simulink model "Tarea4_base"  (R2022b)
settings: Solver=FixedStepDiscrete  StartTime=0.0  StopTime=Tsim  FixedStep=Ts  RelTol=1e-3
values from neighbouring files (symbols this model uses):
  a_adj = ones(3)    [P1.m]
  a_Costo_1 = 0.444    [Tarea4_init.m]
  a_Costo_2 = 0.264    [Tarea4_init.m]
  a_Costo_3 = 0.5    [Tarea4_init.m]
  b_Costo_1 = 0.111    [Tarea4_init.m]
  b_Costo_2 = 0.067    [Tarea4_init.m]
  b_Costo_3 = 0.125    [Tarea4_init.m]
  e_DG1 = 0    [Tarea4_init.m]
  e_DG2 = 0    [Tarea4_init.m]
  e_DG3 = 0    [Tarea4_init.m]
  e_droop = 0    [Tarea4_init.m]
  e_secondary = 100    [Tarea4_init.m]
  fc = 1    [Tarea4_init.m]
  Kii = Lf*wni*wni    (= 8389.16374093)    [Tarea4_init.m]
  Kiv = wnv*wnv*Cf*10    (= 69.0872308076)    [Tarea4_init.m]
  Kpi = 2*zeta*wni*Lf    (= 4.27256600888)    [Tarea4_init.m]
  Kpv = 2*zeta*wnv*Cf*10    (= 0.351858377202)    [Tarea4_init.m]
  Mdc_1 = -30/Pmax_1    (= -0.012)    [Tarea4_init.m]
  Mdc_2 = -30/Pmax_2    (= -0.012)    [Tarea4_init.m]
  Mdc_3 = -30/Pmax_3    (= -0.012)    [Tarea4_init.m]
  mpc_sample_time = 3    [P1.m]
  Pmax_1 = 2500    [Tarea4_init.m]
  Pmax_2 = Pmax_1    (= 2500)    [Tarea4_init.m]
  Pmax_3 = Pmax_1    (= 2500)    [Tarea4_init.m]
  Rl_1_DC = 100    [Tarea4_init.m]
  Rl_2_DC = 100    [Tarea4_init.m]
  Rl_3_DC = 125    [Tarea4_init.m]
  tau = 1*mpc_sample_time    (= 3)    [P1.m]
  Ts = 1/16e3    (= 6.25e-05)    [Tarea4_init.m]
  V0_dc = 400    [Tarea4_init.m]    (also in dmpc.m = parametros(6))
  Vmax_dc = V0_dc+5    (= 405)    [Tarea4_init.m]    (also in dmpc.m = parametros(8))
  Vmin_dc = V0_dc-5    (= 395)    [Tarea4_init.m]    (also in dmpc.m = parametros(7))
undefined symbols (not defined in the file or in its folder): plecs
libraries: slpidlib x6
settings Model: Creator=matib  LastModifiedBy=zanar
settings DebuggingCC: UnconnectedInputMsg=warning  UnconnectedOutputMsg=warning  UnconnectedLineMsg=warning  SFMachineParentedDataDiag=warning  UnderSpecifiedDimensionMsg=warning
settings ModelReferenceCC: EnableRefExpFcnMdlSchedulingChecks=on

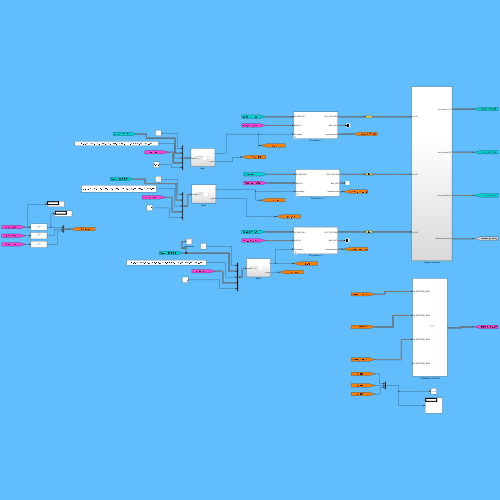
[thumbnail: Simulink's stored preview of the top-level diagram]
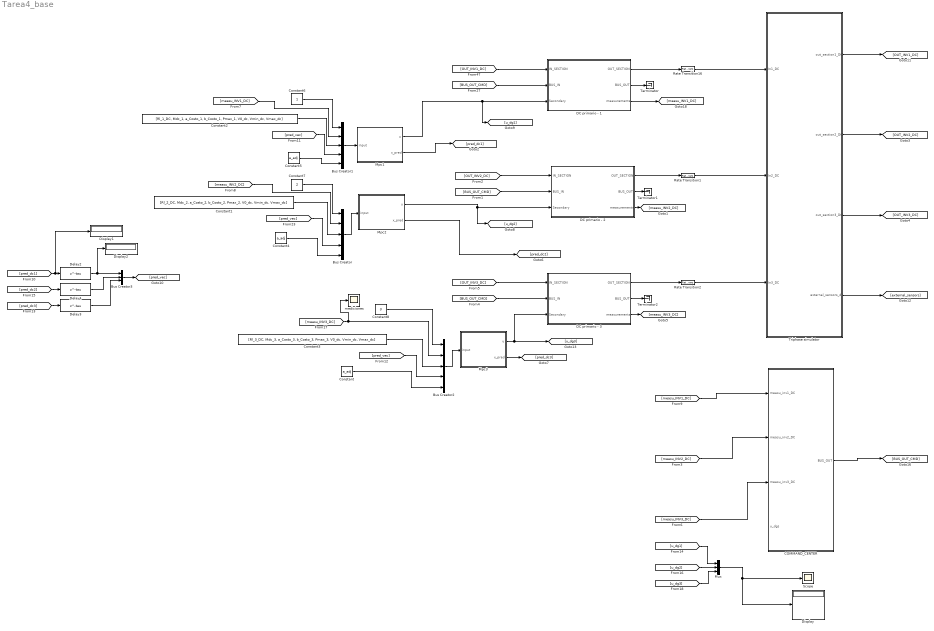
== system Tarea4_base ==
  Bus Creator : BusCreator  Inputs=5
  Bus Creator1 : BusCreator  Inputs=5
  Bus Creator2 : BusCreator  Inputs=5
  Bus Creator3 : BusCreator  Inputs=3
  COMMAND_CENTER : Subsystem
      mask Display:
      | port_label('input', 1, 'IN_SECTION_INV1');
      | port_label('input', 2, 'IN_SECTION_INV2');
      | port_label('input', 3, 'IN_SECTION_INV3');
      | port_label('input', 4, 'IN_SECTION_INV4');
      | 
      | port_label('input', 5, 'MEASUREMENT_INV1');
      | port_label('input', 6, 'MEASUREMENT_INV2');
      | port_label('input', 7, 'MEASUREMENT_INV3');
      | port_label('input', 8, 'MEASUREMENT_INV4');
      | 
      | port_label('input', 9, 'BUS_IN');
      | %port_label('input', 10, 'MEASUREMENT_SECONDARY');
      | 
      | port_label('output', 1, 'BUS_OUT');
  Constant : Constant  Value=a_adj
  Constant1 : Constant  Value=[Rl_2_DC, Mdc_2, a_Costo_2, b_Costo_2, Pmax_2, V0_dc, Vmin_dc, Vmax_dc]
  Constant2 : Constant  Value=[Rl_1_DC, Mdc_1, a_Costo_1, b_Costo_1, Pmax_1, V0_dc, Vmin_dc, Vmax_dc]
  Constant3 : Constant  Value=[Rl_3_DC, Mdc_3, a_Costo_3, b_Costo_3, Pmax_3, V0_dc, Vmin_dc, Vmax_dc]
  Constant4 : Constant  Value=a_adj
  Constant5 : Constant  Value=a_adj
  Constant6 : Constant
  Constant7 : Constant  Value=2
  Constant8 : Constant  Value=3
  DC primario - 1 : Subsystem  mask{Imax=2.5, Pmax=0, Tmax=0}
      mask prompts: Imax "Corriente Máxima"; Pmax "Potencia  Máxima"; Tmax "Temperatura  Máxima"
  DC primario - 2 : Subsystem  mask{Imax=2.5, Pmax=0, Tmax=0}
      mask prompts: Imax "Corriente Máxima"; Pmax "Potencia  Máxima"; Tmax "Temperatura  Máxima"
  DC primario - 3 : Subsystem  mask{Imax=2.5, Pmax=0, Tmax=0}
      mask prompts: Imax "Corriente Máxima"; Pmax "Potencia  Máxima"; Tmax "Temperatura  Máxima"
  Delay2 : Delay  DelayLength=tau
  Delay3 : Delay  DelayLength=tau
  Delay4 : Delay  DelayLength=tau
  Display : Display
  Display1 : Display
  Display2 : Display
  Mpc1 : Subsystem
  Mpc2 : Subsystem
  Mpc3 : Subsystem
  Mux : Mux  Inputs=3
  Rate Transition1 : RateTransition  OutPortSampleTime=Ts
  Rate Transition16 : RateTransition  OutPortSampleTime=Ts
  Rate Transition2 : RateTransition  OutPortSampleTime=Ts
  Scope : Scope
  Terminator : Terminator
  Terminator1 : Terminator
  Terminator2 : Terminator
  Triphase simulator : Subsystem
  mediciones : Scope
  wires:
  Triphase simulator/1(out_section1_DC) -> [OUT_INV1_DC]
  DC primario - 1/1(OUT_SECTION) -> Rate Transition16/1
  Rate Transition16/1 -> Triphase simulator/1(In1_DC)
  [OUT_INV1_DC] -> DC primario - 1/1(IN_SECTION)
  DC primario - 1/3(measurements) -> [measu_INV1_DC]
  [BUS_OUT_CMD] -> DC primario - 1/2(BUS_IN)
  [measu_INV1_DC] -> COMMAND_CENTER/1(measu_inv1_DC)
  COMMAND_CENTER/1(BUS_OUT) -> [BUS_OUT_CMD]
  DC primario - 2/3(measurements) -> [measu_INV2_DC]
  [OUT_INV2_DC] -> DC primario - 2/1(IN_SECTION)
  [BUS_OUT_CMD] -> DC primario - 2/2(BUS_IN)
  DC primario - 2/1(OUT_SECTION) -> Rate Transition1/1
  Rate Transition1/1 -> Triphase simulator/2(In2_DC)
  Triphase simulator/2(out_section2_DC) -> [OUT_INV2_DC]
  [measu_INV2_DC] -> COMMAND_CENTER/2(measu_inv2_DC)
  Triphase simulator/3(out_section3_DC) -> [OUT_INV3_DC]
  Rate Transition2/1 -> Triphase simulator/3(In3_DC)
  DC primario - 3/3(measurements) -> [measu_INV3_DC]
  DC primario - 3/1(OUT_SECTION) -> Rate Transition2/1
  [OUT_INV3_DC] -> DC primario - 3/1(IN_SECTION)
  [BUS_OUT_CMD] -> DC primario - 3/2(BUS_IN)
  [measu_INV3_DC] -> COMMAND_CENTER/3(measu_inv3_DC)
  DC primario - 1/2(BUS_OUT) -> Terminator/1
  DC primario - 2/2(BUS_OUT) -> Terminator1/1
  DC primario - 3/2(BUS_OUT) -> Terminator2/1
  Triphase simulator/4(external_sensors_dc) -> [external_sensors]
  [pred_dc1] -> Display1/1, Delay2/1
  [pred_dc3] -> Delay3/1
  [pred_dc2] -> Delay4/1
  Delay4/1 -> Bus Creator3/2
  Delay3/1 -> Bus Creator3/3
  [pred_vec] -> Bus Creator/4
  Constant1/1 -> Bus Creator/3
  Constant7/1 -> Bus Creator/1
  [measu_INV2_DC] -> Bus Creator/2
  [pred_vec] -> Bus Creator1/4
  [measu_INV1_DC] -> Bus Creator1/2
  Constant2/1 -> Bus Creator1/3
  Constant6/1 -> Bus Creator1/1
  [pred_vec] -> Bus Creator2/4
  Constant8/1 -> Bus Creator2/1
  Constant3/1 -> Bus Creator2/3
  Constant/1 -> Bus Creator2/5
  Constant4/1 -> Bus Creator/5
  Bus Creator3/1 -> [pred_vec]
  Mpc3/1(u) -> [u_dg3], DC primario - 3/3(Secondary)
  Bus Creator2/1 -> Mpc3/1(input)
  [measu_INV3_DC] -> mediciones/1, Bus Creator2/2
  Mpc1/2(x_pred) -> [pred_dc1]
  Mpc1/1(u) -> [u_dg1], DC primario - 1/3(Secondary)
  Bus Creator1/1 -> Mpc1/1(input)
  Bus Creator/1 -> Mpc2/1(input)
  Mpc2/1(u) -> [u_dg2], DC primario - 2/3(Secondary)
  Mpc2/2(x_pred) -> [pred_dc2]
  Mpc3/2(x_pred) -> [pred_dc3]
  Constant5/1 -> Bus Creator1/5
  [u_dg1] -> Mux/1
  [u_dg2] -> Mux/2
  [u_dg3] -> Mux/3
  Mux/1 -> Scope/1, Display/1
  Delay2/1 -> Display2/1, Bus Creator3/1

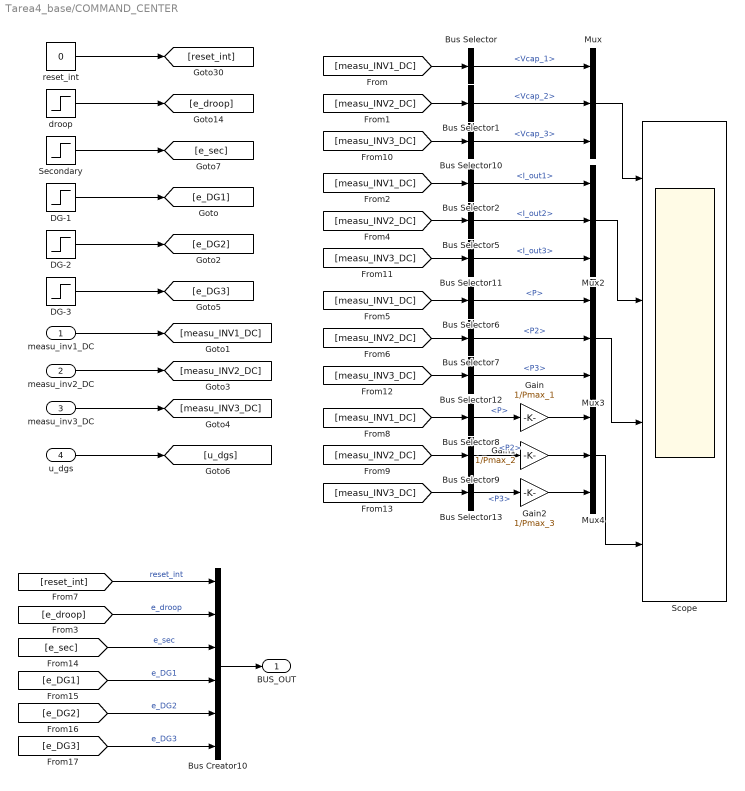
== system Tarea4_base/COMMAND_CENTER ==
  measu_inv1_DC : Inport
  measu_inv2_DC : Inport  Port=2
  measu_inv3_DC : Inport  Port=3
  u_dgs : Inport  Port=4
  Bus Creator10 : BusCreator  Inputs=6
  Bus Selector : BusSelector  OutputSignals=Vcap_1
  Bus Selector1 : BusSelector  OutputSignals=Vcap_2
  Bus Selector10 : BusSelector  OutputSignals=Vcap_3
  Bus Selector11 : BusSelector  OutputSignals=I_out3
  Bus Selector12 : BusSelector  OutputSignals=P3
  Bus Selector13 : BusSelector  OutputSignals=P3
  Bus Selector2 : BusSelector  OutputSignals=I_out1
  Bus Selector5 : BusSelector  OutputSignals=I_out2
  Bus Selector6 : BusSelector  OutputSignals=P
  Bus Selector7 : BusSelector  OutputSignals=P2
  Bus Selector8 : BusSelector  OutputSignals=P
  Bus Selector9 : BusSelector  OutputSignals=P2
  DG-1 : Step  Time=e_DG1  SampleTime=0
  DG-2 : Step  Time=e_DG2  SampleTime=0
  DG-3 : Step  Time=e_DG3  SampleTime=0
  Gain : Gain  Gain=1/Pmax_1
  Gain1 : Gain  Gain=1/Pmax_2
  Gain2 : Gain  Gain=1/Pmax_3
  Mux{,2..4} (4 alike) : Mux  Inputs=3
  Scope : Scope  NumInputPorts=4
  Secondary : Step  Time=e_secondary  SampleTime=0
  droop : Step  Time=e_droop  SampleTime=0
  reset_int : Constant  Value=0  OutDataTypeStr=boolean  SampleTime=Ts
  BUS_OUT : Outport
  wires:
  Bus Creator10/1 -> BUS_OUT/1
  [reset_int] -> Bus Creator10/1  "reset_int"
  reset_int/1 -> [reset_int]
  droop/1 -> [e_droop]
  measu_inv1_DC/1 -> [measu_INV1_DC]
  [e_droop] -> Bus Creator10/2  "e_droop"
  measu_inv2_DC/1 -> [measu_INV2_DC]
  [measu_INV1_DC] -> Bus Selector/1
  [measu_INV2_DC] -> Bus Selector1/1
  Bus Selector1/1 -> Mux/2  "<Vcap_2>"
  Bus Selector/1 -> Mux/1  "<Vcap_1>"
  Bus Selector2/1 -> Mux2/1  "<I_out1>"
  [measu_INV2_DC] -> Bus Selector5/1
  [measu_INV1_DC] -> Bus Selector2/1
  Bus Selector5/1 -> Mux2/2  "<I_out2>"
  [measu_INV1_DC] -> Bus Selector6/1
  Bus Selector7/1 -> Mux3/2  "<P2>"
  [measu_INV2_DC] -> Bus Selector7/1
  Bus Selector6/1 -> Mux3/1  "<P>"
  Mux3/1 -> Scope/3
  Mux2/1 -> Scope/2
  Mux/1 -> Scope/1
  [measu_INV1_DC] -> Bus Selector8/1
  [measu_INV2_DC] -> Bus Selector9/1
  Bus Selector9/1 -> Gain1/1  "<P2>"
  Mux4/1 -> Scope/4
  Bus Selector8/1 -> Gain/1  "<P>"
  Gain/1 -> Mux4/1
  Gain1/1 -> Mux4/2
  measu_inv3_DC/1 -> [measu_INV3_DC]
  Bus Selector10/1 -> Mux/3  "<Vcap_3>"
  [measu_INV3_DC] -> Bus Selector10/1
  [measu_INV3_DC] -> Bus Selector11/1
  Bus Selector11/1 -> Mux2/3  "<I_out3>"
  [measu_INV3_DC] -> Bus Selector12/1
  Bus Selector12/1 -> Mux3/3  "<P3>"
  Bus Selector13/1 -> Gain2/1  "<P3>"
  Gain2/1 -> Mux4/3
  [measu_INV3_DC] -> Bus Selector13/1
  [e_sec] -> Bus Creator10/3  "e_sec"
  [e_DG1] -> Bus Creator10/4  "e_DG1"
  [e_DG2] -> Bus Creator10/5  "e_DG2"
  [e_DG3] -> Bus Creator10/6  "e_DG3"
  DG-1/1 -> [e_DG1]
  DG-2/1 -> [e_DG2]
  DG-3/1 -> [e_DG3]
  Secondary/1 -> [e_sec]
  u_dgs/1 -> [u_dgs]

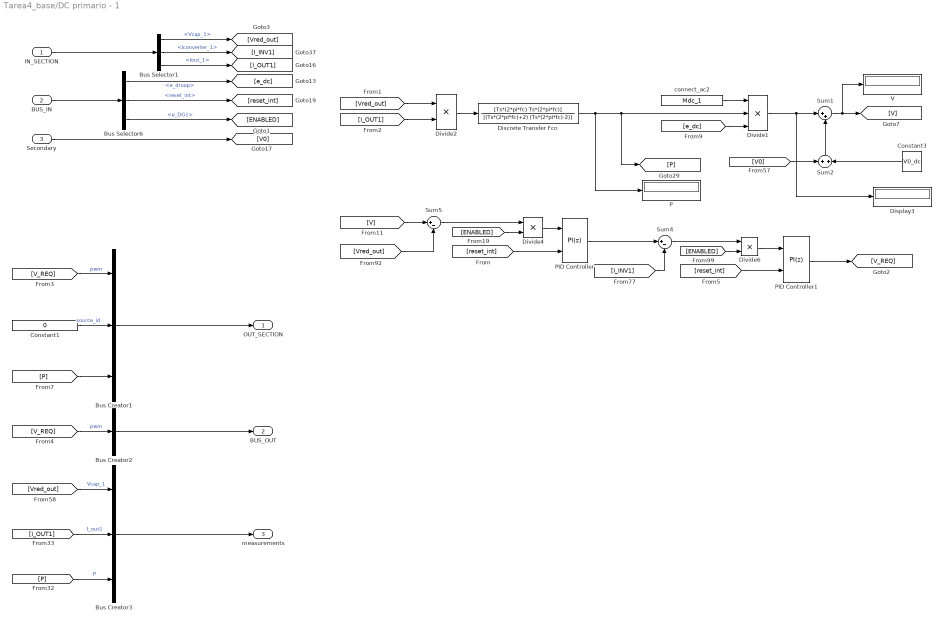
== system Tarea4_base/DC primario - 1 ==
  IN_SECTION : Inport
  BUS_IN : Inport  Port=2
  Secondary : Inport  Port=3
  Bus Creator1 : BusCreator  Inputs=3
  Bus Creator2 : BusCreator  Inputs=1
  Bus Creator3 : BusCreator  Inputs=3
  Bus Selector1 : BusSelector  OutputSignals=Vcap_1,Iconverter_1,Iout_1
  Bus Selector6 : BusSelector  OutputSignals=e_droop,reset_int,e_DG1
  Constant1 : Constant  Value=0  SampleTime=Ts
  Constant3 : Constant  Value=V0_dc  SampleTime=Ts
  Discrete Transfer Fcn : DiscreteTransferFcn  Numerator=[Ts*(2*pi*fc) Ts*(2*pi*fc)]  Denominator=[(Ts*(2*pi*fc)+2) (Ts*(2*pi*fc)-2)]  SampleTime=Ts
  Display3 : Display
  Divide1 : Product  Inputs=3
  Divide2 : Product
  Divide4 : Product  Inputs=**
  Divide6 : Product  Inputs=**
  P : Display
  PID Controller : slpidlib/PID Controller  Controller=PI  Form=Parallel  TimeDomain=Discrete-time  UseExternalTs=off  SampleTime=Ts  IntegratorMethod=Forward Euler  FilterMethod=Forward Euler  ControllerParametersSource=internal  P=Kpv  I=Kiv  UseKiTs=off  D=0  N=100  UseFilter=on  TunerSelectOption=Transfer Function Based (PID Tuner App)  InitialConditionSource=internal  InitialConditionForIntegrator=0  InitialConditionForFilter=0  DifferentiatorICPrevScaledInput=0  ExternalReset=rising  TrackingMode=off  Kt=1  LimitOutput=off  SatLimitsSource=internal  UpperSaturationLimit=500  LowerSaturationLimit=-500  LinearizeAsGain=on  AntiWindupMode=clamping  Kb=1  LimitIntegrator=off  UpperIntegratorSaturationLimit=inf  LowerIntegratorSaturationLimit=-inf  POutMin=[]  POutMax=[]  IOutMin=[]  IOutMax=[]  DOutMin=[]  DOutMax=[]  NOutMin=[]  NOutMax=[]  SumOutMin=[]  SumOutMax=[]  SaturationOutMin=[]  SaturationOutMax=[]  PParamMin=[]  PParamMax=[]  IParamMin=[]  IParamMax=[]  DParamMin=[]  DParamMax=[]  NParamMin=[]  NParamMax=[]  KbParamMin=[]  KbParamMax=[]  KtParamMin=[]  KtParamMax=[]  KbOutMin=[]  KbOutMax=[]  KtOutMin=[]  KtOutMax=[]  IntegratorOutMin=[]  IntegratorOutMax=[]  FilterOutMin=[]  FilterOutMax=[]  SumI1OutMin=[]  SumI1OutMax=[]  SumI2OutMin=[]  SumI2OutMax=[]  SumI3OutMin=[]  SumI3OutMax=[]  SumI4OutMin=[]  SumI4OutMax=[]  SumDOutMin=[]  SumDOutMax=[]  DifferentiatorOutMin=[]  DifferentiatorOutMax=[]  FilterDiffOutCoefMin=[]  FilterDiffOutCoefMax=[]  ReciprocalOutMin=[]  ReciprocalOutMax=[]  SumDenOutMin=[]  SumDenOutMax=[]  SumNumOutMin=[]  SumNumOutMax=[]  DivideOutMin=[]  DivideOutMax=[]  UdiffTsProdOutMin=[]  UdiffTsProdOutMax=[]  NTsProdOutMin=[]  NTsProdOutMax=[]  UintegralTsProdOutMin=[]  UintegralTsProdOutMax=[]  UngainTsProdOutMin=[]  UngainTsProdOutMax=[]  ClampingZeroOutDataTypeStr=Inherit: Inherit via back propagation  ClampingZeroOutMin=[]  ClampingZeroOutMax=[]  FilterDenConstantOutDataTypeStr=Inherit: Inherit via back propagation  FilterDenConstantOutMin=[]  FilterDenConstantOutMax=[]  PCopyOutDataTypeStr=Inherit: Inherit via back propagation  PCopyOutMin=[]  PCopyOutMax=[]  NCopyOutDataTypeStr=Inherit: Inherit via back propagation  NCopyOutMin=[]  NCopyOutMax=[]  IntegratorContinuousStateAttributes=''  IntegratorStateMustResolveToSignalObject=off  IntegratorRTWStateStorageClass=Auto  FilterContinuousStateAttributes=''  FilterStateMustResolveToSignalObject=off  FilterRTWStateStorageClass=Auto  ParallelPVariant=InternalParameters  IdealPVariant=Disabled  IVariant=InternalParameters  DVariant=Disabled  IntegratorVariant=Discrete  SatVariant=Disabled  AWVariant=Passthrough  PCopyVariant=Disabled  TRVariant=Disabled  FdbkBlocksVariant=Forward  IdealPFdbkVariant=Disabled  SatFdbkVariant=Disabled  DerivativeFilterVariant=Disabled  NVariant=Disabled  NCopyVariant=Disabled_SignalSpec  FilterICVariant=Disabled  IntegratorICVariant=InternalICs  ExternalResetVariant=ExternalReset  TRSumVariant=Passthrough  SumFdbkVariant=Disabled  SumVariant=Sum_PI  TsampFilterVariant=InternalTs  TsampNgainVariant=Passthrough  TsampIntegralVariant=Passthrough  ExternalSaturationOutDataTypeStr=Inherit: Same as second input
  PID Controller1 : slpidlib/PID Controller  Controller=PI  Form=Parallel  TimeDomain=Discrete-time  UseExternalTs=off  SampleTime=Ts  IntegratorMethod=Forward Euler  FilterMethod=Forward Euler  ControllerParametersSource=internal  P=Kpi  I=Kii  UseKiTs=off  D=0  N=100  UseFilter=on  TunerSelectOption=Transfer Function Based (PID Tuner App)  InitialConditionSource=internal  InitialConditionForIntegrator=0  InitialConditionForFilter=0  DifferentiatorICPrevScaledInput=0  ExternalReset=rising  TrackingMode=off  Kt=1  LimitOutput=off  SatLimitsSource=internal  UpperSaturationLimit=inf  LowerSaturationLimit=-inf  LinearizeAsGain=on  AntiWindupMode=none  Kb=1  LimitIntegrator=off  UpperIntegratorSaturationLimit=inf  LowerIntegratorSaturationLimit=-inf  POutMin=[]  POutMax=[]  IOutMin=[]  IOutMax=[]  DOutMin=[]  DOutMax=[]  NOutMin=[]  NOutMax=[]  SumOutMin=[]  SumOutMax=[]  SaturationOutMin=[]  SaturationOutMax=[]  PParamMin=[]  PParamMax=[]  IParamMin=[]  IParamMax=[]  DParamMin=[]  DParamMax=[]  NParamMin=[]  NParamMax=[]  KbParamMin=[]  KbParamMax=[]  KtParamMin=[]  KtParamMax=[]  KbOutMin=[]  KbOutMax=[]  KtOutMin=[]  KtOutMax=[]  IntegratorOutMin=[]  IntegratorOutMax=[]  FilterOutMin=[]  FilterOutMax=[]  SumI1OutMin=[]  SumI1OutMax=[]  SumI2OutMin=[]  SumI2OutMax=[]  SumI3OutMin=[]  SumI3OutMax=[]  SumI4OutMin=[]  SumI4OutMax=[]  SumDOutMin=[]  SumDOutMax=[]  DifferentiatorOutMin=[]  DifferentiatorOutMax=[]  FilterDiffOutCoefMin=[]  FilterDiffOutCoefMax=[]  ReciprocalOutMin=[]  ReciprocalOutMax=[]  SumDenOutMin=[]  SumDenOutMax=[]  SumNumOutMin=[]  SumNumOutMax=[]  DivideOutMin=[]  DivideOutMax=[]  UdiffTsProdOutMin=[]  UdiffTsProdOutMax=[]  NTsProdOutMin=[]  NTsProdOutMax=[]  UintegralTsProdOutMin=[]  UintegralTsProdOutMax=[]  UngainTsProdOutMin=[]  UngainTsProdOutMax=[]  ClampingZeroOutDataTypeStr=Inherit: Inherit via back propagation  ClampingZeroOutMin=[]  ClampingZeroOutMax=[]  FilterDenConstantOutDataTypeStr=Inherit: Inherit via back propagation  FilterDenConstantOutMin=[]  FilterDenConstantOutMax=[]  PCopyOutDataTypeStr=Inherit: Inherit via back propagation  PCopyOutMin=[]  PCopyOutMax=[]  NCopyOutDataTypeStr=Inherit: Inherit via back propagation  NCopyOutMin=[]  NCopyOutMax=[]  IntegratorContinuousStateAttributes=''  IntegratorStateMustResolveToSignalObject=off  IntegratorRTWStateStorageClass=Auto  FilterContinuousStateAttributes=''  FilterStateMustResolveToSignalObject=off  FilterRTWStateStorageClass=Auto  ParallelPVariant=InternalParameters  IdealPVariant=Disabled  IVariant=InternalParameters  DVariant=Disabled  IntegratorVariant=Discrete  SatVariant=Disabled  AWVariant=Passthrough  PCopyVariant=Disabled  TRVariant=Disabled  FdbkBlocksVariant=Forward  IdealPFdbkVariant=Disabled  SatFdbkVariant=Disabled  DerivativeFilterVariant=Disabled  NVariant=Disabled  NCopyVariant=Disabled_SignalSpec  FilterICVariant=Disabled  IntegratorICVariant=InternalICs  ExternalResetVariant=ExternalReset  TRSumVariant=Passthrough  SumFdbkVariant=Disabled  SumVariant=Sum_PI  TsampFilterVariant=InternalTs  TsampNgainVariant=Passthrough  TsampIntegralVariant=Passthrough  ExternalSaturationOutDataTypeStr=Inherit: Same as second input
  Sum1 : Sum  Inputs=|++
  Sum2 : Sum  Inputs=+|+
  Sum4 : Sum  Inputs=|+-
  Sum5 : Sum  Inputs=|+-
  V : Display
  connect_ac2 : Constant  Value=Mdc_1  SampleTime=Ts
  OUT_SECTION : Outport  LockScale=on
  BUS_OUT : Outport  Port=2
  measurements : Outport  Port=3
  wires:
  connect_ac2/1 -> Divide1/1
  Sum1/1 -> V/1, [V]
  Divide1/1 -> Display3/1, Sum1/1
  [e_dc] -> Divide1/3
  IN_SECTION/1 -> Bus Selector1/1
  Bus Selector1/2 -> [I_INV1]  "<Iconverter_1>"
  Bus Selector1/3 -> [I_OUT1]  "<Iout_1>"
  Bus Creator2/1 -> BUS_OUT/1
  [V_REQ] -> Bus Creator2/1  "pwm"
  Constant1/1 -> Bus Creator1/2  "source_id"
  Bus Creator1/1 -> OUT_SECTION/1
  Bus Creator3/1 -> measurements/1
  [Vred_out] -> Bus Creator3/1  "Vcap_1"
  [V_REQ] -> Bus Creator1/1  "pwm"
  Sum2/1 -> Sum1/2
  [V0] -> Sum2/1
  [Vred_out] -> Divide2/1
  [I_OUT1] -> Divide2/2
  [P] -> Bus Creator3/3  "P"
  [I_OUT1] -> Bus Creator3/2  "I_out1"
  [P] -> Bus Creator1/3
  Divide2/1 -> Discrete Transfer Fcn/1
  Discrete Transfer Fcn/1 -> Divide1/2, [P], P/1
  Bus Selector1/1 -> [Vred_out]  "<Vcap_1>"
  [Vred_out] -> Sum5/2
  [ENABLED] -> Divide6/2
  [ENABLED] -> Divide4/2
  Sum5/1 -> Divide4/1
  Sum4/1 -> Divide6/1
  [reset_int] -> PID Controller/2
  [V] -> Sum5/1
  [I_INV1] -> Sum4/2
  [reset_int] -> PID Controller1/2
  Divide6/1 -> PID Controller1/1
  Divide4/1 -> PID Controller/1
  PID Controller/1 -> Sum4/1
  Constant3/1 -> Sum2/2
  PID Controller1/1 -> [V_REQ]
  Bus Selector6/2 -> [reset_int]  "<reset_int>"
  Bus Selector6/1 -> [e_dc]  "<e_droop>"
  BUS_IN/1 -> Bus Selector6/1
  Secondary/1 -> [V0]
  Bus Selector6/3 -> [ENABLED]  "<e_DG1>"

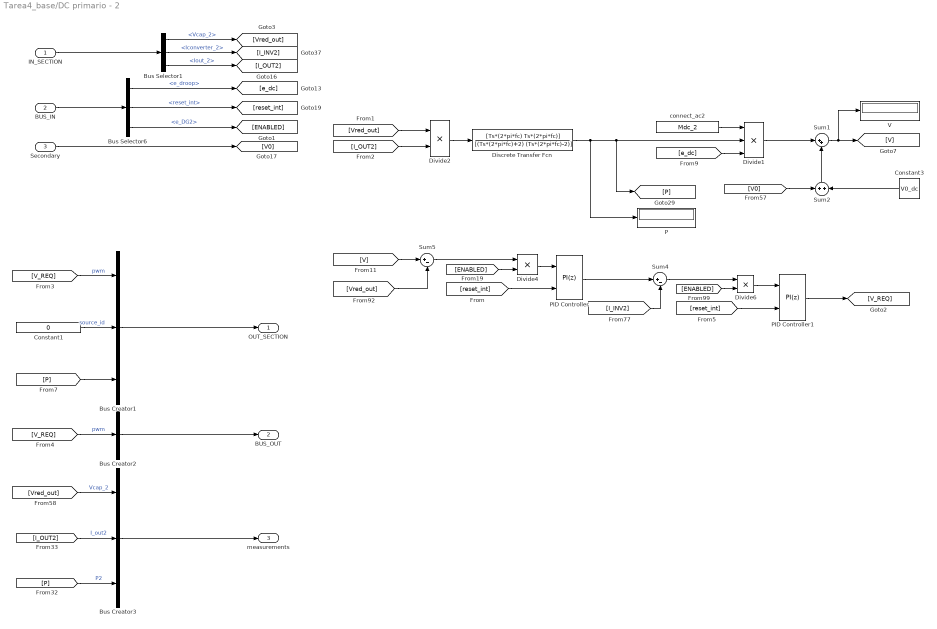
== system Tarea4_base/DC primario - 2 ==
  IN_SECTION : Inport
  BUS_IN : Inport  Port=2
  Secondary : Inport  Port=3
  Bus Creator1 : BusCreator  Inputs=3
  Bus Creator2 : BusCreator  Inputs=1
  Bus Creator3 : BusCreator  Inputs=3
  Bus Selector1 : BusSelector  OutputSignals=Vcap_2,Iconverter_2,Iout_2
  Bus Selector6 : BusSelector  OutputSignals=e_droop,reset_int,e_DG2
  Constant1 : Constant  Value=0  SampleTime=Ts
  Constant3 : Constant  Value=V0_dc  SampleTime=Ts
  Discrete Transfer Fcn : DiscreteTransferFcn  Numerator=[Ts*(2*pi*fc) Ts*(2*pi*fc)]  Denominator=[(Ts*(2*pi*fc)+2) (Ts*(2*pi*fc)-2)]  SampleTime=Ts
  Divide1 : Product  Inputs=3
  Divide2 : Product
  Divide4 : Product  Inputs=**
  Divide6 : Product  Inputs=**
  P : Display
  PID Controller : slpidlib/PID Controller  Controller=PI  Form=Parallel  TimeDomain=Discrete-time  UseExternalTs=off  SampleTime=Ts  IntegratorMethod=Forward Euler  FilterMethod=Forward Euler  ControllerParametersSource=internal  P=Kpv  I=Kiv  UseKiTs=off  D=0  N=100  UseFilter=on  TunerSelectOption=Transfer Function Based (PID Tuner App)  InitialConditionSource=internal  InitialConditionForIntegrator=0  InitialConditionForFilter=0  DifferentiatorICPrevScaledInput=0  ExternalReset=rising  TrackingMode=off  Kt=1  LimitOutput=off  SatLimitsSource=internal  UpperSaturationLimit=500  LowerSaturationLimit=-500  LinearizeAsGain=on  AntiWindupMode=clamping  Kb=1  LimitIntegrator=off  UpperIntegratorSaturationLimit=inf  LowerIntegratorSaturationLimit=-inf  POutMin=[]  POutMax=[]  IOutMin=[]  IOutMax=[]  DOutMin=[]  DOutMax=[]  NOutMin=[]  NOutMax=[]  SumOutMin=[]  SumOutMax=[]  SaturationOutMin=[]  SaturationOutMax=[]  PParamMin=[]  PParamMax=[]  IParamMin=[]  IParamMax=[]  DParamMin=[]  DParamMax=[]  NParamMin=[]  NParamMax=[]  KbParamMin=[]  KbParamMax=[]  KtParamMin=[]  KtParamMax=[]  KbOutMin=[]  KbOutMax=[]  KtOutMin=[]  KtOutMax=[]  IntegratorOutMin=[]  IntegratorOutMax=[]  FilterOutMin=[]  FilterOutMax=[]  SumI1OutMin=[]  SumI1OutMax=[]  SumI2OutMin=[]  SumI2OutMax=[]  SumI3OutMin=[]  SumI3OutMax=[]  SumI4OutMin=[]  SumI4OutMax=[]  SumDOutMin=[]  SumDOutMax=[]  DifferentiatorOutMin=[]  DifferentiatorOutMax=[]  FilterDiffOutCoefMin=[]  FilterDiffOutCoefMax=[]  ReciprocalOutMin=[]  ReciprocalOutMax=[]  SumDenOutMin=[]  SumDenOutMax=[]  SumNumOutMin=[]  SumNumOutMax=[]  DivideOutMin=[]  DivideOutMax=[]  UdiffTsProdOutMin=[]  UdiffTsProdOutMax=[]  NTsProdOutMin=[]  NTsProdOutMax=[]  UintegralTsProdOutMin=[]  UintegralTsProdOutMax=[]  UngainTsProdOutMin=[]  UngainTsProdOutMax=[]  ClampingZeroOutDataTypeStr=Inherit: Inherit via back propagation  ClampingZeroOutMin=[]  ClampingZeroOutMax=[]  FilterDenConstantOutDataTypeStr=Inherit: Inherit via back propagation  FilterDenConstantOutMin=[]  FilterDenConstantOutMax=[]  PCopyOutDataTypeStr=Inherit: Inherit via back propagation  PCopyOutMin=[]  PCopyOutMax=[]  NCopyOutDataTypeStr=Inherit: Inherit via back propagation  NCopyOutMin=[]  NCopyOutMax=[]  IntegratorContinuousStateAttributes=''  IntegratorStateMustResolveToSignalObject=off  IntegratorRTWStateStorageClass=Auto  FilterContinuousStateAttributes=''  FilterStateMustResolveToSignalObject=off  FilterRTWStateStorageClass=Auto  ParallelPVariant=InternalParameters  IdealPVariant=Disabled  IVariant=InternalParameters  DVariant=Disabled  IntegratorVariant=Discrete  SatVariant=Disabled  AWVariant=Passthrough  PCopyVariant=Disabled  TRVariant=Disabled  FdbkBlocksVariant=Forward  IdealPFdbkVariant=Disabled  SatFdbkVariant=Disabled  DerivativeFilterVariant=Disabled  NVariant=Disabled  NCopyVariant=Disabled_SignalSpec  FilterICVariant=Disabled  IntegratorICVariant=InternalICs  ExternalResetVariant=ExternalReset  TRSumVariant=Passthrough  SumFdbkVariant=Disabled  SumVariant=Sum_PI  TsampFilterVariant=InternalTs  TsampNgainVariant=Passthrough  TsampIntegralVariant=Passthrough  ExternalSaturationOutDataTypeStr=Inherit: Same as second input
  PID Controller1 : slpidlib/PID Controller  Controller=PI  Form=Parallel  TimeDomain=Discrete-time  UseExternalTs=off  SampleTime=Ts  IntegratorMethod=Forward Euler  FilterMethod=Forward Euler  ControllerParametersSource=internal  P=Kpi  I=Kii  UseKiTs=off  D=0  N=100  UseFilter=on  TunerSelectOption=Transfer Function Based (PID Tuner App)  InitialConditionSource=internal  InitialConditionForIntegrator=0  InitialConditionForFilter=0  DifferentiatorICPrevScaledInput=0  ExternalReset=rising  TrackingMode=off  Kt=1  LimitOutput=off  SatLimitsSource=internal  UpperSaturationLimit=inf  LowerSaturationLimit=-inf  LinearizeAsGain=on  AntiWindupMode=none  Kb=1  LimitIntegrator=off  UpperIntegratorSaturationLimit=inf  LowerIntegratorSaturationLimit=-inf  POutMin=[]  POutMax=[]  IOutMin=[]  IOutMax=[]  DOutMin=[]  DOutMax=[]  NOutMin=[]  NOutMax=[]  SumOutMin=[]  SumOutMax=[]  SaturationOutMin=[]  SaturationOutMax=[]  PParamMin=[]  PParamMax=[]  IParamMin=[]  IParamMax=[]  DParamMin=[]  DParamMax=[]  NParamMin=[]  NParamMax=[]  KbParamMin=[]  KbParamMax=[]  KtParamMin=[]  KtParamMax=[]  KbOutMin=[]  KbOutMax=[]  KtOutMin=[]  KtOutMax=[]  IntegratorOutMin=[]  IntegratorOutMax=[]  FilterOutMin=[]  FilterOutMax=[]  SumI1OutMin=[]  SumI1OutMax=[]  SumI2OutMin=[]  SumI2OutMax=[]  SumI3OutMin=[]  SumI3OutMax=[]  SumI4OutMin=[]  SumI4OutMax=[]  SumDOutMin=[]  SumDOutMax=[]  DifferentiatorOutMin=[]  DifferentiatorOutMax=[]  FilterDiffOutCoefMin=[]  FilterDiffOutCoefMax=[]  ReciprocalOutMin=[]  ReciprocalOutMax=[]  SumDenOutMin=[]  SumDenOutMax=[]  SumNumOutMin=[]  SumNumOutMax=[]  DivideOutMin=[]  DivideOutMax=[]  UdiffTsProdOutMin=[]  UdiffTsProdOutMax=[]  NTsProdOutMin=[]  NTsProdOutMax=[]  UintegralTsProdOutMin=[]  UintegralTsProdOutMax=[]  UngainTsProdOutMin=[]  UngainTsProdOutMax=[]  ClampingZeroOutDataTypeStr=Inherit: Inherit via back propagation  ClampingZeroOutMin=[]  ClampingZeroOutMax=[]  FilterDenConstantOutDataTypeStr=Inherit: Inherit via back propagation  FilterDenConstantOutMin=[]  FilterDenConstantOutMax=[]  PCopyOutDataTypeStr=Inherit: Inherit via back propagation  PCopyOutMin=[]  PCopyOutMax=[]  NCopyOutDataTypeStr=Inherit: Inherit via back propagation  NCopyOutMin=[]  NCopyOutMax=[]  IntegratorContinuousStateAttributes=''  IntegratorStateMustResolveToSignalObject=off  IntegratorRTWStateStorageClass=Auto  FilterContinuousStateAttributes=''  FilterStateMustResolveToSignalObject=off  FilterRTWStateStorageClass=Auto  ParallelPVariant=InternalParameters  IdealPVariant=Disabled  IVariant=InternalParameters  DVariant=Disabled  IntegratorVariant=Discrete  SatVariant=Disabled  AWVariant=Passthrough  PCopyVariant=Disabled  TRVariant=Disabled  FdbkBlocksVariant=Forward  IdealPFdbkVariant=Disabled  SatFdbkVariant=Disabled  DerivativeFilterVariant=Disabled  NVariant=Disabled  NCopyVariant=Disabled_SignalSpec  FilterICVariant=Disabled  IntegratorICVariant=InternalICs  ExternalResetVariant=ExternalReset  TRSumVariant=Passthrough  SumFdbkVariant=Disabled  SumVariant=Sum_PI  TsampFilterVariant=InternalTs  TsampNgainVariant=Passthrough  TsampIntegralVariant=Passthrough  ExternalSaturationOutDataTypeStr=Inherit: Same as second input
  Sum1 : Sum  Inputs=|++
  Sum2 : Sum  Inputs=+|+
  Sum4 : Sum  Inputs=|+-
  Sum5 : Sum  Inputs=|+-
  V : Display
  connect_ac2 : Constant  Value=Mdc_2  SampleTime=Ts
  OUT_SECTION : Outport  LockScale=on
  BUS_OUT : Outport  Port=2
  measurements : Outport  Port=3
  wires:
  IN_SECTION/1 -> Bus Selector1/1
  Bus Selector1/2 -> [I_INV2]  "<Iconverter_2>"
  Bus Selector1/3 -> [I_OUT2]  "<Iout_2>"
  Bus Creator2/1 -> BUS_OUT/1
  [V_REQ] -> Bus Creator2/1  "pwm"
  Constant1/1 -> Bus Creator1/2  "source_id"
  Bus Creator1/1 -> OUT_SECTION/1
  Bus Creator3/1 -> measurements/1
  [Vred_out] -> Bus Creator3/1  "Vcap_2"
  [V_REQ] -> Bus Creator1/1  "pwm"
  [P] -> Bus Creator3/3  "P2"
  [I_OUT2] -> Bus Creator3/2  "I_out2"
  [P] -> Bus Creator1/3
  Bus Selector1/1 -> [Vred_out]  "<Vcap_2>"
  Divide2/1 -> Discrete Transfer Fcn/1
  connect_ac2/1 -> Divide1/1
  Sum1/1 -> V/1, [V]
  Discrete Transfer Fcn/1 -> Divide1/2, [P], P/1
  [V0] -> Sum2/1
  Divide1/1 -> Sum1/1
  Sum2/1 -> Sum1/2
  Constant3/1 -> Sum2/2
  [e_dc] -> Divide1/3
  [Vred_out] -> Divide2/1
  [I_OUT2] -> Divide2/2
  Sum4/1 -> Divide6/1
  [reset_int] -> PID Controller/2
  [ENABLED] -> Divide4/2
  Divide6/1 -> PID Controller1/1
  [Vred_out] -> Sum5/2
  Sum5/1 -> Divide4/1
  [reset_int] -> PID Controller1/2
  [I_INV2] -> Sum4/2
  Divide4/1 -> PID Controller/1
  [V] -> Sum5/1
  PID Controller1/1 -> [V_REQ]
  [ENABLED] -> Divide6/2
  PID Controller/1 -> Sum4/1
  Bus Selector6/2 -> [reset_int]  "<reset_int>"
  Bus Selector6/1 -> [e_dc]  "<e_droop>"
  Secondary/1 -> [V0]
  BUS_IN/1 -> Bus Selector6/1
  Bus Selector6/3 -> [ENABLED]  "<e_DG2>"

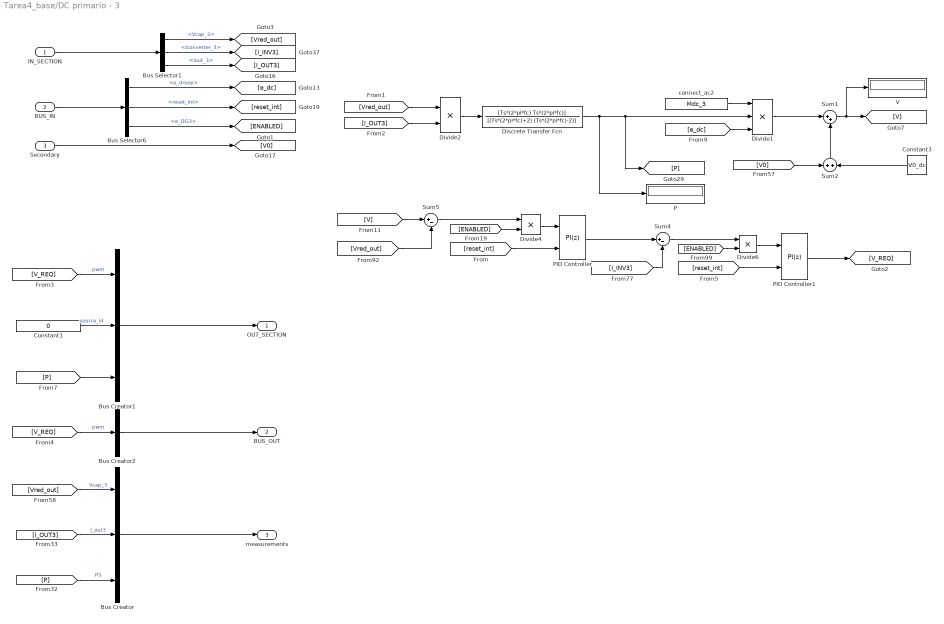
== system Tarea4_base/DC primario - 3 ==
  IN_SECTION : Inport
  BUS_IN : Inport  Port=2
  Secondary : Inport  Port=3
  Bus Creator : BusCreator  Inputs=3
  Bus Creator1 : BusCreator  Inputs=3
  Bus Creator2 : BusCreator  Inputs=1
  Bus Selector1 : BusSelector  OutputSignals=Vcap_3,Iconverter_3,Iout_3
  Bus Selector6 : BusSelector  OutputSignals=e_droop,reset_int,e_DG3
  Constant1 : Constant  Value=0  SampleTime=Ts
  Constant3 : Constant  Value=V0_dc  SampleTime=Ts
  Discrete Transfer Fcn : DiscreteTransferFcn  Numerator=[Ts*(2*pi*fc) Ts*(2*pi*fc)]  Denominator=[(Ts*(2*pi*fc)+2) (Ts*(2*pi*fc)-2)]  SampleTime=Ts
  Divide1 : Product  Inputs=3
  Divide2 : Product
  Divide4 : Product  Inputs=**
  Divide6 : Product  Inputs=**
  P : Display
  PID Controller : slpidlib/PID Controller  Controller=PI  Form=Parallel  TimeDomain=Discrete-time  UseExternalTs=off  SampleTime=Ts  IntegratorMethod=Forward Euler  FilterMethod=Forward Euler  ControllerParametersSource=internal  P=Kpv  I=Kiv  UseKiTs=off  D=0  N=100  UseFilter=on  TunerSelectOption=Transfer Function Based (PID Tuner App)  InitialConditionSource=internal  InitialConditionForIntegrator=0  InitialConditionForFilter=0  DifferentiatorICPrevScaledInput=0  ExternalReset=rising  TrackingMode=off  Kt=1  LimitOutput=off  SatLimitsSource=internal  UpperSaturationLimit=500  LowerSaturationLimit=-500  LinearizeAsGain=on  AntiWindupMode=clamping  Kb=1  LimitIntegrator=off  UpperIntegratorSaturationLimit=inf  LowerIntegratorSaturationLimit=-inf  POutMin=[]  POutMax=[]  IOutMin=[]  IOutMax=[]  DOutMin=[]  DOutMax=[]  NOutMin=[]  NOutMax=[]  SumOutMin=[]  SumOutMax=[]  SaturationOutMin=[]  SaturationOutMax=[]  PParamMin=[]  PParamMax=[]  IParamMin=[]  IParamMax=[]  DParamMin=[]  DParamMax=[]  NParamMin=[]  NParamMax=[]  KbParamMin=[]  KbParamMax=[]  KtParamMin=[]  KtParamMax=[]  KbOutMin=[]  KbOutMax=[]  KtOutMin=[]  KtOutMax=[]  IntegratorOutMin=[]  IntegratorOutMax=[]  FilterOutMin=[]  FilterOutMax=[]  SumI1OutMin=[]  SumI1OutMax=[]  SumI2OutMin=[]  SumI2OutMax=[]  SumI3OutMin=[]  SumI3OutMax=[]  SumI4OutMin=[]  SumI4OutMax=[]  SumDOutMin=[]  SumDOutMax=[]  DifferentiatorOutMin=[]  DifferentiatorOutMax=[]  FilterDiffOutCoefMin=[]  FilterDiffOutCoefMax=[]  ReciprocalOutMin=[]  ReciprocalOutMax=[]  SumDenOutMin=[]  SumDenOutMax=[]  SumNumOutMin=[]  SumNumOutMax=[]  DivideOutMin=[]  DivideOutMax=[]  UdiffTsProdOutMin=[]  UdiffTsProdOutMax=[]  NTsProdOutMin=[]  NTsProdOutMax=[]  UintegralTsProdOutMin=[]  UintegralTsProdOutMax=[]  UngainTsProdOutMin=[]  UngainTsProdOutMax=[]  ClampingZeroOutDataTypeStr=Inherit: Inherit via back propagation  ClampingZeroOutMin=[]  ClampingZeroOutMax=[]  FilterDenConstantOutDataTypeStr=Inherit: Inherit via back propagation  FilterDenConstantOutMin=[]  FilterDenConstantOutMax=[]  PCopyOutDataTypeStr=Inherit: Inherit via back propagation  PCopyOutMin=[]  PCopyOutMax=[]  NCopyOutDataTypeStr=Inherit: Inherit via back propagation  NCopyOutMin=[]  NCopyOutMax=[]  IntegratorContinuousStateAttributes=''  IntegratorStateMustResolveToSignalObject=off  IntegratorRTWStateStorageClass=Auto  FilterContinuousStateAttributes=''  FilterStateMustResolveToSignalObject=off  FilterRTWStateStorageClass=Auto  ParallelPVariant=InternalParameters  IdealPVariant=Disabled  IVariant=InternalParameters  DVariant=Disabled  IntegratorVariant=Discrete  SatVariant=Disabled  AWVariant=Passthrough  PCopyVariant=Disabled  TRVariant=Disabled  FdbkBlocksVariant=Forward  IdealPFdbkVariant=Disabled  SatFdbkVariant=Disabled  DerivativeFilterVariant=Disabled  NVariant=Disabled  NCopyVariant=Disabled_SignalSpec  FilterICVariant=Disabled  IntegratorICVariant=InternalICs  ExternalResetVariant=ExternalReset  TRSumVariant=Passthrough  SumFdbkVariant=Disabled  SumVariant=Sum_PI  TsampFilterVariant=InternalTs  TsampNgainVariant=Passthrough  TsampIntegralVariant=Passthrough  ExternalSaturationOutDataTypeStr=Inherit: Same as second input
  PID Controller1 : slpidlib/PID Controller  Controller=PI  Form=Parallel  TimeDomain=Discrete-time  UseExternalTs=off  SampleTime=Ts  IntegratorMethod=Forward Euler  FilterMethod=Forward Euler  ControllerParametersSource=internal  P=Kpi  I=Kii  UseKiTs=off  D=0  N=100  UseFilter=on  TunerSelectOption=Transfer Function Based (PID Tuner App)  InitialConditionSource=internal  InitialConditionForIntegrator=0  InitialConditionForFilter=0  DifferentiatorICPrevScaledInput=0  ExternalReset=rising  TrackingMode=off  Kt=1  LimitOutput=off  SatLimitsSource=internal  UpperSaturationLimit=inf  LowerSaturationLimit=-inf  LinearizeAsGain=on  AntiWindupMode=none  Kb=1  LimitIntegrator=off  UpperIntegratorSaturationLimit=inf  LowerIntegratorSaturationLimit=-inf  POutMin=[]  POutMax=[]  IOutMin=[]  IOutMax=[]  DOutMin=[]  DOutMax=[]  NOutMin=[]  NOutMax=[]  SumOutMin=[]  SumOutMax=[]  SaturationOutMin=[]  SaturationOutMax=[]  PParamMin=[]  PParamMax=[]  IParamMin=[]  IParamMax=[]  DParamMin=[]  DParamMax=[]  NParamMin=[]  NParamMax=[]  KbParamMin=[]  KbParamMax=[]  KtParamMin=[]  KtParamMax=[]  KbOutMin=[]  KbOutMax=[]  KtOutMin=[]  KtOutMax=[]  IntegratorOutMin=[]  IntegratorOutMax=[]  FilterOutMin=[]  FilterOutMax=[]  SumI1OutMin=[]  SumI1OutMax=[]  SumI2OutMin=[]  SumI2OutMax=[]  SumI3OutMin=[]  SumI3OutMax=[]  SumI4OutMin=[]  SumI4OutMax=[]  SumDOutMin=[]  SumDOutMax=[]  DifferentiatorOutMin=[]  DifferentiatorOutMax=[]  FilterDiffOutCoefMin=[]  FilterDiffOutCoefMax=[]  ReciprocalOutMin=[]  ReciprocalOutMax=[]  SumDenOutMin=[]  SumDenOutMax=[]  SumNumOutMin=[]  SumNumOutMax=[]  DivideOutMin=[]  DivideOutMax=[]  UdiffTsProdOutMin=[]  UdiffTsProdOutMax=[]  NTsProdOutMin=[]  NTsProdOutMax=[]  UintegralTsProdOutMin=[]  UintegralTsProdOutMax=[]  UngainTsProdOutMin=[]  UngainTsProdOutMax=[]  ClampingZeroOutDataTypeStr=Inherit: Inherit via back propagation  ClampingZeroOutMin=[]  ClampingZeroOutMax=[]  FilterDenConstantOutDataTypeStr=Inherit: Inherit via back propagation  FilterDenConstantOutMin=[]  FilterDenConstantOutMax=[]  PCopyOutDataTypeStr=Inherit: Inherit via back propagation  PCopyOutMin=[]  PCopyOutMax=[]  NCopyOutDataTypeStr=Inherit: Inherit via back propagation  NCopyOutMin=[]  NCopyOutMax=[]  IntegratorContinuousStateAttributes=''  IntegratorStateMustResolveToSignalObject=off  IntegratorRTWStateStorageClass=Auto  FilterContinuousStateAttributes=''  FilterStateMustResolveToSignalObject=off  FilterRTWStateStorageClass=Auto  ParallelPVariant=InternalParameters  IdealPVariant=Disabled  IVariant=InternalParameters  DVariant=Disabled  IntegratorVariant=Discrete  SatVariant=Disabled  AWVariant=Passthrough  PCopyVariant=Disabled  TRVariant=Disabled  FdbkBlocksVariant=Forward  IdealPFdbkVariant=Disabled  SatFdbkVariant=Disabled  DerivativeFilterVariant=Disabled  NVariant=Disabled  NCopyVariant=Disabled_SignalSpec  FilterICVariant=Disabled  IntegratorICVariant=InternalICs  ExternalResetVariant=ExternalReset  TRSumVariant=Passthrough  SumFdbkVariant=Disabled  SumVariant=Sum_PI  TsampFilterVariant=InternalTs  TsampNgainVariant=Passthrough  TsampIntegralVariant=Passthrough  ExternalSaturationOutDataTypeStr=Inherit: Same as second input
  Sum1 : Sum  Inputs=|++
  Sum2 : Sum  Inputs=+|+
  Sum4 : Sum  Inputs=|+-
  Sum5 : Sum  Inputs=|+-
  V : Display
  connect_ac2 : Constant  Value=Mdc_3  SampleTime=Ts
  OUT_SECTION : Outport  LockScale=on
  BUS_OUT : Outport  Port=2
  measurements : Outport  Port=3
  wires:
  IN_SECTION/1 -> Bus Selector1/1
  Bus Selector1/2 -> [I_INV3]  "<Iconverter_3>"
  Bus Selector1/3 -> [I_OUT3]  "<Iout_3>"
  Bus Creator2/1 -> BUS_OUT/1
  [V_REQ] -> Bus Creator2/1  "pwm"
  Constant1/1 -> Bus Creator1/2  "source_id"
  Bus Creator1/1 -> OUT_SECTION/1
  [Vred_out] -> Bus Creator/1  "Vcap_3"
  [V_REQ] -> Bus Creator1/1  "pwm"
  [P] -> Bus Creator/3  "P3"
  [I_OUT3] -> Bus Creator/2  "I_out3"
  [P] -> Bus Creator1/3
  Bus Selector1/1 -> [Vred_out]  "<Vcap_3>"
  Bus Creator/1 -> measurements/1
  Divide2/1 -> Discrete Transfer Fcn/1
  connect_ac2/1 -> Divide1/1
  Sum1/1 -> V/1, [V]
  Discrete Transfer Fcn/1 -> Divide1/2, [P], P/1
  [V0] -> Sum2/1
  Divide1/1 -> Sum1/1
  Sum2/1 -> Sum1/2
  Constant3/1 -> Sum2/2
  [e_dc] -> Divide1/3
  [Vred_out] -> Divide2/1
  [I_OUT3] -> Divide2/2
  Sum4/1 -> Divide6/1
  [reset_int] -> PID Controller/2
  [ENABLED] -> Divide4/2
  Divide6/1 -> PID Controller1/1
  [Vred_out] -> Sum5/2
  Sum5/1 -> Divide4/1
  [reset_int] -> PID Controller1/2
  [I_INV3] -> Sum4/2
  Divide4/1 -> PID Controller/1
  [V] -> Sum5/1
  PID Controller1/1 -> [V_REQ]
  [ENABLED] -> Divide6/2
  PID Controller/1 -> Sum4/1
  Bus Selector6/2 -> [reset_int]  "<reset_int>"
  Bus Selector6/1 -> [e_dc]  "<e_droop>"
  Secondary/1 -> [V0]
  BUS_IN/1 -> Bus Selector6/1
  Bus Selector6/3 -> [ENABLED]  "<e_DG3>"

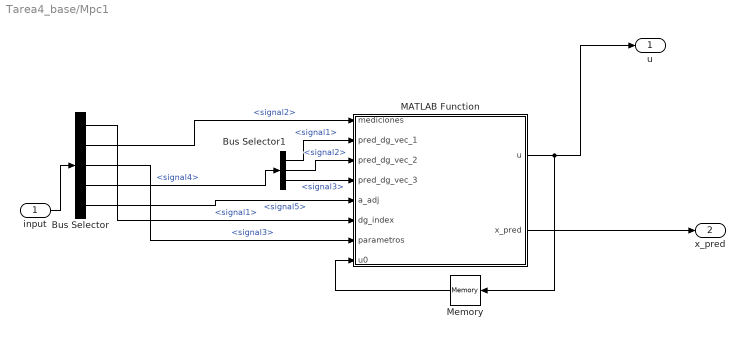
== system Tarea4_base/Mpc1 ==
  input : Inport
  Bus Selector : BusSelector  OutputSignals=signal1,signal2,signal3,signal4,signal5
  Bus Selector1 : BusSelector  OutputSignals=signal1,signal2,signal3
  MATLAB Function : MATLAB Function  TreatAsAtomicUnit=on  SystemSampleTime=mpc_sample_time
      settings: MinAlgLoopOccurrences=on
  Memory : Memory
  u : Outport
  x_pred : Outport  Port=2
  wires:
  MATLAB Function/1(u) -> Memory/1, u/1
  input/1 -> Bus Selector/1
  Bus Selector/2 -> MATLAB Function/1(mediciones)  "<signal2>"
  Bus Selector/4 -> Bus Selector1/1  "<signal4>"
  Bus Selector1/1 -> MATLAB Function/2(pred_dg_vec_1)  "<signal1>"
  Bus Selector1/2 -> MATLAB Function/3(pred_dg_vec_2)  "<signal2>"
  Bus Selector1/3 -> MATLAB Function/4(pred_dg_vec_3)  "<signal3>"
  MATLAB Function/2(x_pred) -> x_pred/1
  Bus Selector/1 -> MATLAB Function/6(dg_index)  "<signal1>"
  Bus Selector/3 -> MATLAB Function/7(parametros)  "<signal3>"
  Bus Selector/5 -> MATLAB Function/5(a_adj)  "<signal5>"
  Memory/1 -> MATLAB Function/8(u0)

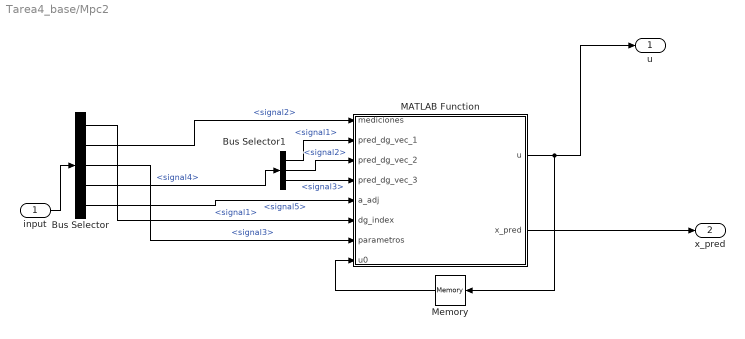
== system Tarea4_base/Mpc2 ==
  input : Inport
  Bus Selector : BusSelector  OutputSignals=signal1,signal2,signal3,signal4,signal5
  Bus Selector1 : BusSelector  OutputSignals=signal1,signal2,signal3
  MATLAB Function : MATLAB Function  TreatAsAtomicUnit=on  SystemSampleTime=mpc_sample_time
      settings: MinAlgLoopOccurrences=on
  Memory : Memory
  u : Outport
  x_pred : Outport  Port=2
  wires:
  Bus Selector/5 -> MATLAB Function/5(a_adj)  "<signal5>"
  Bus Selector/3 -> MATLAB Function/7(parametros)  "<signal3>"
  Bus Selector/1 -> MATLAB Function/6(dg_index)  "<signal1>"
  MATLAB Function/2(x_pred) -> x_pred/1
  Bus Selector1/3 -> MATLAB Function/4(pred_dg_vec_3)  "<signal3>"
  Bus Selector1/2 -> MATLAB Function/3(pred_dg_vec_2)  "<signal2>"
  Bus Selector1/1 -> MATLAB Function/2(pred_dg_vec_1)  "<signal1>"
  Bus Selector/4 -> Bus Selector1/1  "<signal4>"
  Bus Selector/2 -> MATLAB Function/1(mediciones)  "<signal2>"
  input/1 -> Bus Selector/1
  MATLAB Function/1(u) -> u/1, Memory/1
  Memory/1 -> MATLAB Function/8(u0)

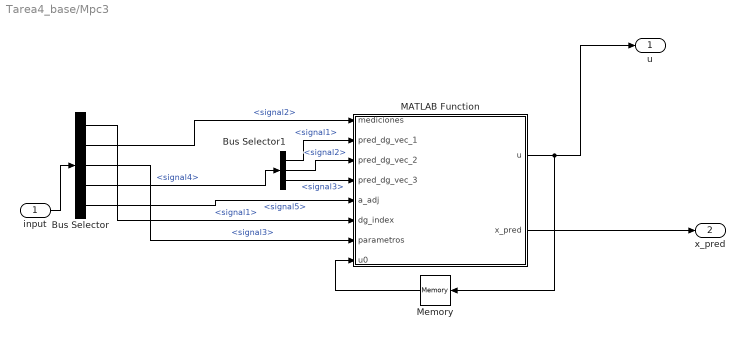
== system Tarea4_base/Mpc3 ==
  input : Inport
  Bus Selector : BusSelector  OutputSignals=signal1,signal2,signal3,signal4,signal5
  Bus Selector1 : BusSelector  OutputSignals=signal1,signal2,signal3
  MATLAB Function : MATLAB Function  TreatAsAtomicUnit=on  SystemSampleTime=mpc_sample_time
      settings: MinAlgLoopOccurrences=on
  Memory : Memory
  u : Outport
  x_pred : Outport  Port=2
  wires:
  MATLAB Function/1(u) -> Memory/1, u/1
  input/1 -> Bus Selector/1
  Bus Selector/2 -> MATLAB Function/1(mediciones)  "<signal2>"
  Bus Selector/4 -> Bus Selector1/1  "<signal4>"
  Bus Selector1/1 -> MATLAB Function/2(pred_dg_vec_1)  "<signal1>"
  Bus Selector1/2 -> MATLAB Function/3(pred_dg_vec_2)  "<signal2>"
  Bus Selector1/3 -> MATLAB Function/4(pred_dg_vec_3)  "<signal3>"
  MATLAB Function/2(x_pred) -> x_pred/1
  Bus Selector/1 -> MATLAB Function/6(dg_index)  "<signal1>"
  Bus Selector/3 -> MATLAB Function/7(parametros)  "<signal3>"
  Bus Selector/5 -> MATLAB Function/5(a_adj)  "<signal5>"
  Memory/1 -> MATLAB Function/8(u0)

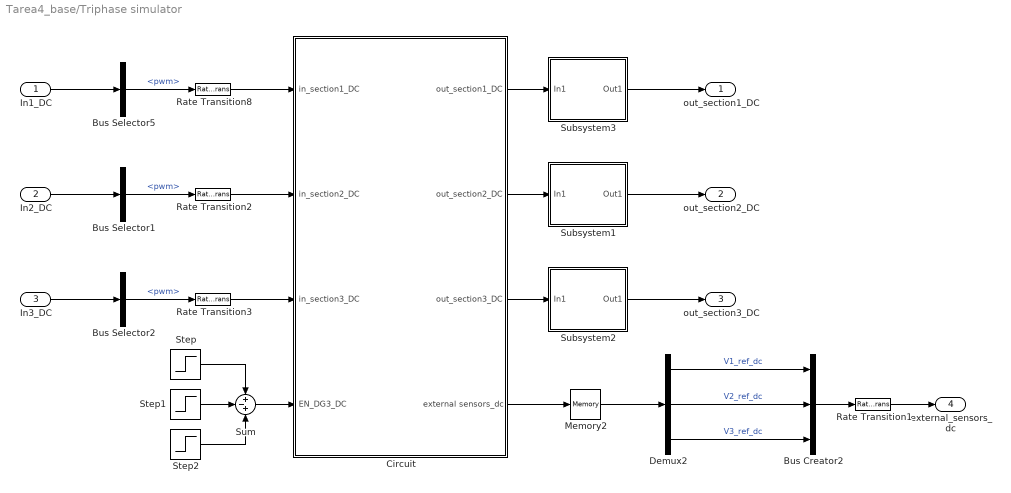
== system Tarea4_base/Triphase simulator ==
  In1_DC : Inport
  In2_DC : Inport  Port=2
  In3_DC : Inport  Port=3
  Bus Creator2 : BusCreator  Inputs=3
  Bus Selector1 : BusSelector  OutputSignals=pwm
  Bus Selector2 : BusSelector  OutputSignals=pwm
  Bus Selector5 : BusSelector  OutputSignals=pwm
  Circuit : Subsystem  LoadFcn=plecs('sl', 200);  InitFcn=plecs('sl', 214);  StartFcn=plecs('sl', 208);  StopFcn=plecs('sl', 209);  mask(PlecsCircuit){PLECSData=<binary blob, 7112 chars, not shown>}
      mask prompts: PLECSData "PLECS Data (Do not delete or modify!)"
      mask init:
      | % PLACE CUSTOM INITIALIZATIONS ABOVE
      | % DO NOT REMOVE
      | plecs('sl', 215);
      | % DO NOT REMOVE
      settings: CopyFcn=plecs('sl', 203);  DeleteFcn=plecs('sl', 205);  UndoDeleteFcn=plecs('sl', 206);  PreSaveFcn=plecs('sl', 211);  PostSaveFcn=plecs('sl', 201);  NameChangeFcn=plecs('sl', 210);  DestroyFcn=plecs('sl', 207);  PreCopyFcn=plecs('sl', 216);  OpenFcn=plecs('sl', 202);  ErrorFcn=plerrorfcn
      mask Help: eval('plecs(''help'', ''qthelp:///creatingacircuit.html'')')
      mask Display: disp('PLECS\nCircuit')
  Demux2 : Demux  Outputs=[1 1 1]
  Memory2 : Memory
  Rate Transition{1..3,8} (4 alike) : RateTransition  OutPortSampleTime=Ts
  Step : Step  Time=10  SampleTime=Ts
  Step1 : Step  Time=37  SampleTime=Ts
  Step2 : Step  Time=45  SampleTime=Ts
  Subsystem1 : Subsystem
  Subsystem2 : Subsystem
  Subsystem3 : Subsystem
  Sum : Sum  Inputs=+-+
  out_section1_DC : Outport
  out_section2_DC : Outport  Port=2
  out_section3_DC : Outport  Port=3
  external_sensors_dc : Outport  Port=4
  wires:
  Rate Transition1/1 -> external_sensors_dc/1
  Demux2/2 -> Bus Creator2/2  "V2_ref_dc"
  Demux2/1 -> Bus Creator2/1  "V1_ref_dc"
  Memory2/1 -> Demux2/1
  Bus Creator2/1 -> Rate Transition1/1
  Demux2/3 -> Bus Creator2/3  "V3_ref_dc"
  Circuit/4(external sensors_dc) -> Memory2/1
  Subsystem3/1(Out1) -> out_section1_DC/1
  Circuit/1(out_section1_DC) -> Subsystem3/1(In1)
  In1_DC/1 -> Bus Selector5/1
  Bus Selector5/1 -> Rate Transition8/1  "<pwm>"
  Rate Transition8/1 -> Circuit/1(in_section1_DC)
  In2_DC/1 -> Bus Selector1/1
  Bus Selector1/1 -> Rate Transition2/1  "<pwm>"
  Rate Transition2/1 -> Circuit/2(in_section2_DC)
  Circuit/2(out_section2_DC) -> Subsystem1/1(In1)
  Subsystem1/1(Out1) -> out_section2_DC/1
  Subsystem2/1(Out1) -> out_section3_DC/1
  Circuit/3(out_section3_DC) -> Subsystem2/1(In1)
  In3_DC/1 -> Bus Selector2/1
  Rate Transition3/1 -> Circuit/3(in_section3_DC)
  Bus Selector2/1 -> Rate Transition3/1  "<pwm>"
  Step/1 -> Sum/1
  Sum/1 -> Circuit/4(EN_DG3_DC)
  Step1/1 -> Sum/2
  Step2/1 -> Sum/3

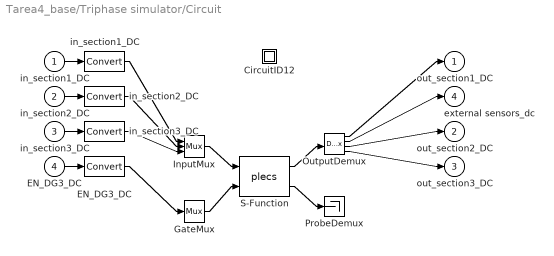
== system Tarea4_base/Triphase simulator/Circuit ==
  in_section1_DC : Inport  PortDimensions=1
  in_section2_DC : Inport  Port=2  PortDimensions=1
  in_section3_DC : Inport  Port=3  PortDimensions=1
  EN_DG3_DC : Inport  Port=4  PortDimensions=1
  " CircuitID12 " : Subsystem
  " EN_DG3_DC " : DataTypeConversion
  " GateMux " : Mux  Inputs=[ 1 ]
  " InputMux " : Mux  Inputs=[ 1 1 1 ]
  " OutputDemux " : Demux  Outputs=[ 3 3 3 3 ]
  " ProbeDemux " : Terminator
  " S-Function " : S-Function  FunctionName=plecs  SFunctionDeploymentMode=off  EnableBusSupport=off
  " in_section1_DC " : DataTypeConversion
  " in_section2_DC " : DataTypeConversion
  " in_section3_DC " : DataTypeConversion
  out_section1_DC : Outport  PortDimensions=3
  out_section2_DC : Outport  Port=2  PortDimensions=3
  out_section3_DC : Outport  Port=3  PortDimensions=3
  external sensors_dc : Outport  Port=4  PortDimensions=3
  wires:
  " InputMux "/1 -> " S-Function "/1
  " GateMux "/1 -> " S-Function "/2
  " S-Function "/1 -> " OutputDemux "/1
  " S-Function "/2 -> " ProbeDemux "/1
  in_section1_DC/1 -> " in_section1_DC "/1
  " in_section1_DC "/1 -> " InputMux "/1
  in_section2_DC/1 -> " in_section2_DC "/1
  " in_section2_DC "/1 -> " InputMux "/2
  in_section3_DC/1 -> " in_section3_DC "/1
  " in_section3_DC "/1 -> " InputMux "/3
  EN_DG3_DC/1 -> " EN_DG3_DC "/1
  " EN_DG3_DC "/1 -> " GateMux "/1
  " OutputDemux "/1 -> out_section1_DC/1
  " OutputDemux "/2 -> external sensors_dc/1
  " OutputDemux "/3 -> out_section2_DC/1
  " OutputDemux "/4 -> out_section3_DC/1

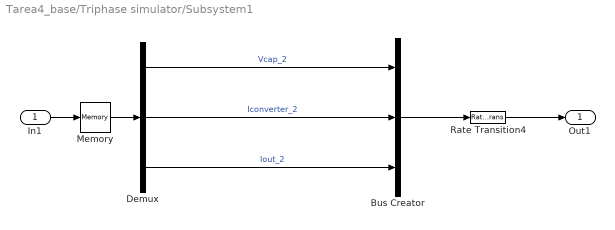
== system Tarea4_base/Triphase simulator/Subsystem1 ==
  In1 : Inport
  Bus Creator : BusCreator  Inputs=3
  Demux : Demux  Outputs=[1 1 1]
  Memory : Memory
  Rate Transition4 : RateTransition  OutPortSampleTime=Ts
  Out1 : Outport
  wires:
  Bus Creator/1 -> Rate Transition4/1
  In1/1 -> Memory/1
  Memory/1 -> Demux/1
  Rate Transition4/1 -> Out1/1
  Demux/1 -> Bus Creator/1  "Vcap_2"
  Demux/2 -> Bus Creator/2  "Iconverter_2"
  Demux/3 -> Bus Creator/3  "Iout_2"

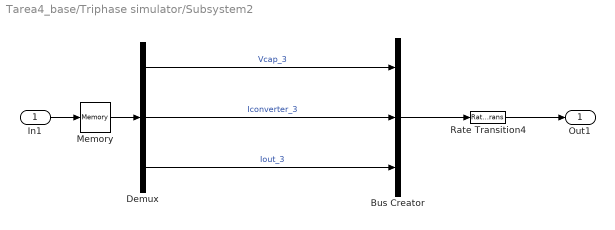
== system Tarea4_base/Triphase simulator/Subsystem2 ==
  In1 : Inport
  Bus Creator : BusCreator  Inputs=3
  Demux : Demux  Outputs=[1 1 1]
  Memory : Memory
  Rate Transition4 : RateTransition  OutPortSampleTime=Ts
  Out1 : Outport
  wires:
  Bus Creator/1 -> Rate Transition4/1
  In1/1 -> Memory/1
  Memory/1 -> Demux/1
  Rate Transition4/1 -> Out1/1
  Demux/1 -> Bus Creator/1  "Vcap_3"
  Demux/2 -> Bus Creator/2  "Iconverter_3"
  Demux/3 -> Bus Creator/3  "Iout_3"

== system Tarea4_base/Triphase simulator/Subsystem3 ==
  In1 : Inport
  Bus Creator : BusCreator  Inputs=3
  Demux : Demux  Outputs=[1 1 1]
  Memory : Memory
  Rate Transition4 : RateTransition  OutPortSampleTime=Ts
  Out1 : Outport
  wires:
  Bus Creator/1 -> Rate Transition4/1
  In1/1 -> Memory/1
  Memory/1 -> Demux/1
  Rate Transition4/1 -> Out1/1
  Demux/1 -> Bus Creator/1  "Vcap_1"
  Demux/2 -> Bus Creator/2  "Iconverter_1"
  Demux/3 -> Bus Creator/3  "Iout_1"

== system Tarea4_base/Triphase simulator/Circuit/ CircuitID12  ==

== matlab function Tarea4_base/Mpc2/MATLAB Function ==
  data: u output; x_pred output; mediciones input size=3; pred_dg_vec_1 input; pred_dg_vec_2 input; pred_dg_vec_3 input; parametros_mpc parameter; a_adj input; dg_index input; parametros input; u0 input
function [u, x_pred] = fcn(mediciones, pred_dg_vec_1, pred_dg_vec_2, pred_dg_vec_3, parametros_mpc, a_adj, dg_index, parametros, u0)
u=0;

[accion_control, pred_mpc] = dmpc(dg_index, mediciones, parametros, [pred_dg_vec_1, pred_dg_vec_2 pred_dg_vec_3], a_adj, parametros_mpc, u0);

u = u + accion_control;
x_pred = pred_mpc;
end

== matlab function Tarea4_base/Mpc3/MATLAB Function ==
  data: u output; x_pred output; mediciones input size=3; pred_dg_vec_1 input; pred_dg_vec_2 input; pred_dg_vec_3 input; parametros_mpc parameter; a_adj input; dg_index input; parametros input; u0 input
function [u, x_pred] = fcn(mediciones, pred_dg_vec_1, pred_dg_vec_2, pred_dg_vec_3, parametros_mpc, a_adj, dg_index, parametros, u0)
u=0;

[accion_control, pred_mpc] = dmpc(dg_index, mediciones, parametros, [pred_dg_vec_1, pred_dg_vec_2 pred_dg_vec_3], a_adj, parametros_mpc, u0);

u = u + accion_control;
x_pred = pred_mpc;
end

== matlab function Tarea4_base/Mpc1/MATLAB Function ==
  data: u output; x_pred output; mediciones input size=3; pred_dg_vec_1 input; pred_dg_vec_2 input; pred_dg_vec_3 input; parametros_mpc parameter; a_adj input; dg_index input; parametros input; u0 input
function [u, x_pred] = fcn(mediciones, pred_dg_vec_1, pred_dg_vec_2, pred_dg_vec_3, parametros_mpc, a_adj, dg_index, parametros, u0)
u=0;

[accion_control, pred_mpc] = dmpc(dg_index, mediciones, parametros, [pred_dg_vec_1, pred_dg_vec_2 pred_dg_vec_3], a_adj, parametros_mpc, u0);

u = u + accion_control;
x_pred = pred_mpc;
end
